simulink model "Vehicle_Control_CodeGen"  (R2024a)
settings: Solver=FixedStepAuto  StartTime=0.0  StopTime=10  RelTol=1e-3  EnableMultiTasking=on
undefined symbols (not defined in the file or in its folder): CAN, DiscIntNeverNeededParam, FD, Ion, Lithium
libraries: stmutilitieslib x28, simulink x21, stm32blockslib x10, canfdmsglib x6, dspstat3 x6, slpidlib x3, spsBatteryLib x2, spsControlledCurrentSourceLib x2, spsVoltageMeasurementLib x2, spspowerguiLib x2, stm32h7xxblockslib x2
(part 3 of 3)

== system Vehicle_Control_CodeGen/Variant Subsystem/CAN Forwarding ==
  In1 : Inport
  Out1 : Outport
  wires:
  In1/1 -> Out1/1

== system Vehicle_Control_CodeGen/Variant Subsystem/Simulation of Throttle Pedal ==
  note: Set sim time to 2154
  note: Throttle Input
  Constant1 : Constant  Value=50
  Constant25 : Constant  Value=100
  From File : FromFile  FileName=endurancedata.mat  SampleTime=0.1
  Manual Switch2 : ManualSwitch  CurrentSetting=0
  Product8 : Product
  Scope12 : Scope
  Out1 : Outport
  wires:
  From File/1 -> Product8/1  "Throttle"
  Constant1/1 -> Manual Switch2/1  "Throttle Percentage"
  Product8/1 -> Scope12/1, Manual Switch2/2  "Throttle"
  Constant25/1 -> Product8/2
  Manual Switch2/1 -> Out1/1

== system Vehicle_Control_CodeGen/Variant Subsystem1/Battery Model1 ==
  note: Delay increased to 3 x 0.01 second to test robustness. This is to simulate the delay of having voltage measurments sent to the VCU
  note: Battery Model is from SIM SCAPE Tool box. Uses a constant current drive to take the current request from controller and apply load to the battery
  Requested Current : Inport
  Battery1 : spsBatteryLib/Battery  BatType=Lithium-Ion  ShowTempParam=off  ThermalPreset=no  ShowAgeParam=off  NomV=532.8  NomQ=1152  SOC=85  Batt_Tr=5  PresetModel=on  MaxQ=1152  MinV=399.6  FullV=620.1723  Dis_rate=500.8696  R=0.004625  Normal_OP=1041.8087  expZone="[575.6296      56.59826]"  current=[6.5 13 32.5]  Units=Time  Tci=20  NomT=20  T2=-30  MaxQ2=4.8  FullV2=7.1  Normal_OP2=5.655  expZone2="[6.58           1]"  Rca=0.6  ti=2000  Dp=0  Neq0=0  Tsim=1e6  Ta1=25  Qeol=5.4*0.9  Reol=0.013333*1.2  Char_age=[2.3478, 3]  Dis_age=[2.3478, 10]  N1=1500  N2=10500  N3=1000  N4=1400  Ta2=45  N5=950
  Controlled Current Source1 : spsControlledCurrentSourceLib/Controlled Current Source  Initialize=on  Source_Type=AC  Amplitude=0  Phase=0  Frequency=0  Measurements=None
  Delay2 : Delay  DelayLength=5  InitialCondition=580
  Scope5 : Scope
  Voltage Measurement1 : spsVoltageMeasurementLib/Voltage Measurement  PhasorSimulation=off  OutputType=Complex  PSBequivalent=0
  powergui1 : spspowerguiLib/powergui  Priority=1  SimulationMode=Discrete  SampleTime=0.001  frequency=60  Iterations=50  frequencyindice=0  Pbase=100e6  ErrMax=1e-4  UnitsV=kV  UnitsW=MW  buscounter=0  FunctionMessages=off  echomessages=off  EnableUseOfTLC=off  CurrentSourceSwitches=off  DisableSnubberDevices=off  DisableRonSwitches=off  DisableVfSwitches=off  DisplayEquations=off  AutomaticDiscreteSolvers=off  SolverType=Tustin/Backward Euler (TBE)  Interpol=off  ExternalGateDelay=off  methode=off  Ts=100  x0status=blocks  SPID=on  SwTol=0  HookPort=off  NonlinearTolerance=1e-4  nMaxIteration=100  ContinueOnMaxIteration=off  RestoreLinks=warning  ResistiveCurrentMeasurement=off  Frange=[0:2:500]  Ylog=off  Xlog=on  ShowGrid=off  save=off  variable=ZData  structure=0  ZoomFFT=off  StartTime=0.0  cycles=1  DisplayStyle=1  fundamental=60  FreqAxis=off  MaxFrequency=1000  frequencyindicesteady=1  RmsSteady=1  display=off
  Scope : Outport
  Batt Out : Outport  Port=2
  wires:
  Voltage Measurement1/1 -> Delay2/1, Scope/1, Scope5/1  "BUS Voltage"
  Requested Current/1 -> Controlled Current Source1/1
  Delay2/1 -> Batt Out/1  "Batter Voltage"
  Battery1/1 -> ?
  connections:
  Voltage Measurement1/LConn1 -- Controlled Current Source1/RConn1 -- Battery1/LConn1
  Battery1/LConn2 -- Voltage Measurement1/LConn2 -- Controlled Current Source1/LConn1

== system Vehicle_Control_CodeGen/Variant Subsystem1/CAN Forwarding ==
  Can Sig : Inport
  Batt Out : Outport
  Scope : Outport  Port=2
  wires:
  Can Sig/1 -> Scope/1, Batt Out/1

== system Vehicle_Control_CodeGen/Power Forcasting/Variant Subsystem/CAN Forwarding ==
  CAN SOC : Inport
  Out1 : Outport
  wires:
  CAN SOC/1 -> Out1/1

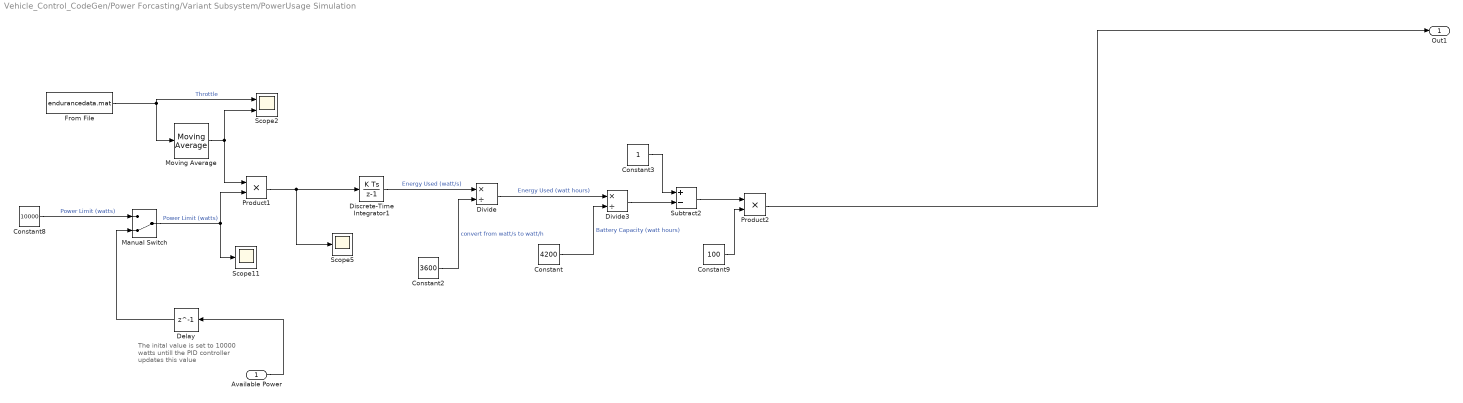
== system Vehicle_Control_CodeGen/Power Forcasting/Variant Subsystem/PowerUsage Simulation ==
  note: The inital value is set to 10000 watts untill the PID controller updates this value
  Available Power : Inport
  Constant : Constant  Value=4200
  Constant2 : Constant  Value=3600
  Constant3 : Constant
  Constant8 : Constant  Value=10000
  Constant9 : Constant  Value=100
  Delay : Delay  DelayLength=1  InitialCondition=10000
  Discrete-Time Integrator1 : DiscreteIntegrator  SampleTime=-1  ICPrevOutput=DiscIntNeverNeededParam  ICPrevScaledInput=DiscIntNeverNeededParam
  Divide : Product  Inputs=*/
  Divide3 : Product  Inputs=*/
  From File : FromFile  FileName=endurancedata.mat
  Manual Switch : ManualSwitch  CurrentSetting=0
  Moving Average : dspstat3/Moving Average  Method=Sliding window  ForgettingFactorPort=off  SpecifyWindowLength=on  WindowLength=1000  OverlapLength=999  AllowArbitraryInputLength=off  ForgettingFactor=0.9  SimulateUsing=Interpreted execution
  Product1 : Product
  Product2 : Product
  Scope11 : Scope
  Scope2 : Scope  NumInputPorts=2
  Scope5 : Scope
  Subtract2 : Sum  Inputs=+-
  Out1 : Outport
  wires:
  Moving Average/1 -> Scope2/2, Product1/1
  Constant8/1 -> Manual Switch/1  "Power Limit (watts)"
  Divide/1 -> Divide3/1  "Energy Used (watt hours)"
  Product1/1 -> Scope5/1, Discrete-Time Integrator1/1
  Divide3/1 -> Subtract2/2
  Delay/1 -> Manual Switch/2
  Subtract2/1 -> Product2/1
  Manual Switch/1 -> Scope11/1, Product1/2  "Power Limit (watts)"
  Constant9/1 -> Product2/2
  From File/1 -> Scope2/1, Moving Average/1  "Throttle"
  Discrete-Time Integrator1/1 -> Divide/1  "Energy Used (watt/s)"
  Constant3/1 -> Subtract2/1
  Constant2/1 -> Divide/2  "convert from watt/s to watt/h"
  Constant/1 -> Divide3/2  "Battery Capacity (watt hours)"
  Product2/1 -> Out1/1
  Available Power/1 -> Delay/1

== system Vehicle_Control_CodeGen/Power Forcasting/Variant Subsystem1/Code Gen, Wheel speed averaging and integration ==
  note: Filtering input to try and stop large changes in rate of change of distance traveled
  In2 : Inport
  In1 : Inport  Port=2
  Add2 : Sum
  Constant2 : Constant  Value=2
  Discrete-Time Integrator2 : DiscreteIntegrator  SampleTime=-1  ICPrevOutput=DiscIntNeverNeededParam  ICPrevScaledInput=DiscIntNeverNeededParam
  Divide : Product  Inputs=*/
  Moving Average1 : dspstat3/Moving Average  Method=Sliding window  ForgettingFactorPort=off  SpecifyWindowLength=on  WindowLength=1000  OverlapLength=999  AllowArbitraryInputLength=off  ForgettingFactor=0.9  SimulateUsing=Interpreted execution
  Scope : Scope
  Scope1 : Scope
  1 : Outport
  wires:
  Constant2/1 -> Divide/2
  Add2/1 -> Divide/1
  Divide/1 -> Discrete-Time Integrator2/1  "Average Speed"
  In2/1 -> Add2/1  "Right Wheel Speed"
  In1/1 -> Scope/1, Add2/2  "Left Wheel Speed"
  Discrete-Time Integrator2/1 -> Moving Average1/1  "Distance Traveled"
  Moving Average1/1 -> Scope1/1, 1/1

== system Vehicle_Control_CodeGen/Power Forcasting/Variant Subsystem1/Fake wheel speed from simulation ==
  note: Filtering input to try and stop large changes in rate of change of distance traveled
  Add2 : Sum
  Constant1 : Constant  Value=2
  Discrete-Time Integrator2 : DiscreteIntegrator  SampleTime=-1  ICPrevOutput=DiscIntNeverNeededParam  ICPrevScaledInput=DiscIntNeverNeededParam
  Discrete-Time Integrator3 : DiscreteIntegrator  SampleTime=-1  ICPrevOutput=DiscIntNeverNeededParam  ICPrevScaledInput=DiscIntNeverNeededParam
  Divide2 : Product  Inputs=*/
  From File1 : FromFile  FileName=simspeed.mat
  From File2 : FromFile  FileName=simspeed.mat
  From File3 : FromFile  FileName=simspeed.mat
  Manual Switch2 : ManualSwitch  CurrentSetting=0
  Moving Average1 : dspstat3/Moving Average  Method=Sliding window  ForgettingFactorPort=off  SpecifyWindowLength=on  WindowLength=1000  OverlapLength=999  AllowArbitraryInputLength=off  ForgettingFactor=0.9  SimulateUsing=Interpreted execution
  Moving Average2 : dspstat3/Moving Average  Method=Sliding window  ForgettingFactorPort=off  SpecifyWindowLength=on  WindowLength=1000  OverlapLength=999  AllowArbitraryInputLength=off  ForgettingFactor=0.9  SimulateUsing=Interpreted execution
  Scope : Scope
  Scope7 : Scope
  Scope8 : Scope  NumInputPorts=2
  Scope9 : Scope
  1 : Outport
  wires:
  Constant1/1 -> Divide2/2
  From File3/1 -> Add2/1  "Right Wheel Speed"
  Add2/1 -> Divide2/1
  Discrete-Time Integrator3/1 -> Moving Average2/1  "Distance Traveled"
  From File1/1 -> Scope7/1, Discrete-Time Integrator2/1  "vehicle Speed"
  Divide2/1 -> Discrete-Time Integrator3/1  "Average Speed"
  Discrete-Time Integrator2/1 -> Scope8/2, Moving Average1/1  "Distance Traveled"
  Moving Average2/1 -> Manual Switch2/1, Scope9/1  "Distance Traveled"
  Moving Average1/1 -> Scope8/1, Manual Switch2/2
  From File2/1 -> Scope/1, Add2/2  "Left Wheel Speed"
  Manual Switch2/1 -> 1/1

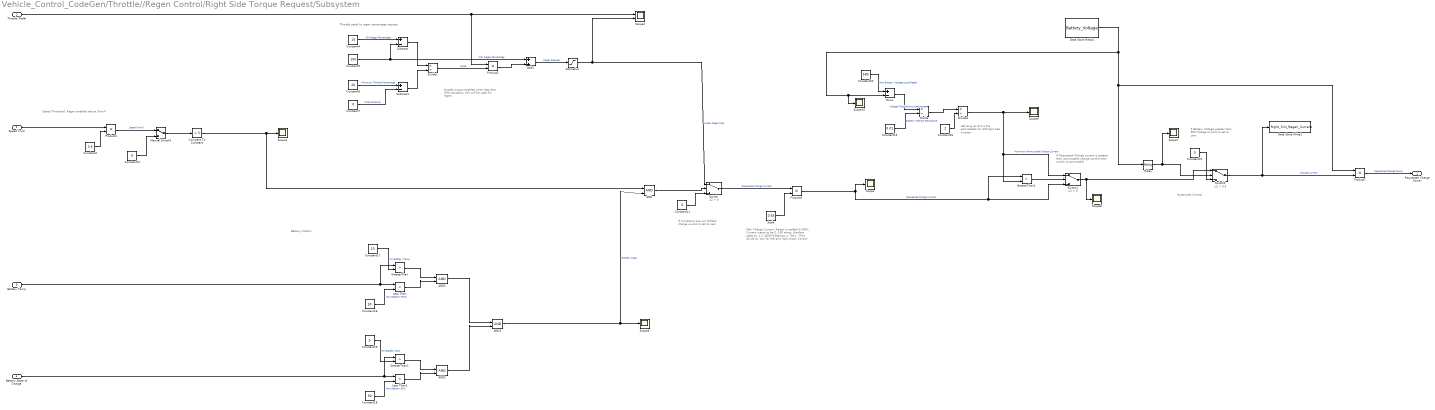
== system Vehicle_Control_CodeGen/Throttle//Regen Control/Right Side Torque Request/Subsystem ==
  note: Halveing as this is the permissable for left/right side inverter
  note: If Conditions are not fulfilled charge current is set to zero
  note: Throttle pedal to regen percentage request
  note: throttle output enabled when less then 20% actuation, this will be used for regen
  note: If Battery Voltage greater then 590 Charge Current is set to zero
  note: Speed Threshold, Regen enabled above 5km/h
  note: Max Charge Current, Regen is scalled 0-100%. Current wants to be 0 -130 amps, therfore scale by 1.3. 600V*130amps = 70kw, Then divide by two for left and right motor Control
  note: Hysterisies Control
  note: Battery Checks
  note: If Requested Charge current is greater then permissable charge current then switch to permisable
  Throttle Pedal : Inport
  Speed (m/s) : Inport  Port=2
  Battery Temp : Inport  Port=3
  Battery State of Charge : Inport  Port=4
  AND{,1..3} (4 alike) : Logic  IconShape=distinctive  AllPortsSameDT=off  OutDataTypeStr=boolean
  Add3 : Sum
  Compare To Constant : simulink/Logic and Bit Operations/Compare To Constant  relop=>  const=5  OutDataTypeStr=boolean
  Constant11 : Constant  Value=0
  Constant12 : Constant  Value=6
  Constant15 : Constant  Value=0.01
  Constant16 : Constant  Value=50
  Constant17 : Constant  Value=10
  Constant18 : Constant  Value=90
  Constant19 : Constant  Value=5
  Constant2 : Constant  Value=3.6
  Constant20 : Constant  Value=580
  Constant21 : Constant  Value=0
  Constant26 : Constant  Value=2
  Constant4 : Constant  Value=10
  Constant5 : Constant  Value=100
  Constant6 : Constant  Value=20
  Constant7 : Constant  Value=0
  Data Store Read1 : DataStoreRead  DataStoreName=Battery_Voltage  IndexOptions=Index vector (dialog)  Indices=1  OutputSizes=1
  Data Store Write1 : DataStoreWrite  DataStoreName=Right_Sim_Regen_Current  IndexOptions=Index vector (dialog)  Indices=1  OutputSizes=1
  Divide : Product  Inputs=*/
  Divide1 : Product  Inputs=*/
  Divide4 : Product  Inputs=*/
  GreaterThan : RelationalOperator  Operator=>  OutDataTypeStr=boolean  RndMeth=Simplest  InputSameDT=off
  GreaterThan1 : RelationalOperator  Operator=>  OutDataTypeStr=boolean  RndMeth=Simplest  InputSameDT=off
  GreaterThan2 : RelationalOperator  Operator=>  OutDataTypeStr=boolean  RndMeth=Simplest  InputSameDT=off
  Less Than : RelationalOperator  Operator=<  OutDataTypeStr=boolean  RndMeth=Simplest  InputSameDT=off
  Less Than1 : RelationalOperator  Operator=<  OutDataTypeStr=boolean  RndMeth=Simplest  InputSameDT=off
  Manual Switch1 : ManualSwitch
  Minus : Sum  Inputs=+-
  Product{1..2,4,7} (4 alike) : Product
  Relay : Relay  OnSwitchValue=590  OffSwitchValue=585  OnOutputValue=0  OffOutputValue=1
  Saturation : Saturate  UpperLimit=100  LowerLimit=0
  Scale : Constant  Value=0.65
  Scope{,1,3,7..9,15} (7 alike) : Scope
  Scope2 : Scope  NumInputPorts=2
  Subtract : Sum  Inputs=+-
  Subtract1 : Sum  Inputs=+-
  Switch : Switch  Criteria=u2 > Threshold  SaturateOnIntegerOverflow=off  InputSameDT=off
  Switch1 : Switch  Criteria=u2 > Threshold  SaturateOnIntegerOverflow=off  InputSameDT=off
  Switch2 : Switch  Criteria=u2 > Threshold  Threshold=0.5  SaturateOnIntegerOverflow=off  InputSameDT=off
  Requested Charge Power : Outport
  wires:
  AND3/1 -> Scope3/1, AND/2  "Battery Logic"
  Constant21/1 -> Switch2/3
  Constant5/1 -> Subtract/2, Add3/1  "Max Regen Percentage"
  Relay/1 -> Switch2/2, Scope7/1
  Manual Switch1/1 -> Compare To Constant/1
  Constant2/1 -> Product1/2
  Constant18/1 -> Less Than1/2  "Max Battery SOC"
  Constant20/1 -> Minus/1  "Max Battery Voltage using Regen"
  Compare To Constant/1 -> AND/1, Scope1/1
  Subtract1/1 -> Divide1/2
  Divide1/1 -> Product2/2  "Slope"
  Constant12/1 -> Manual Switch1/2
  Scale/1 -> Product4/2
  Constant17/1 -> GreaterThan/2  "Min Battery Temp"
  Constant16/1 -> Less Than/2  "Max Battery temp"
  Throttle Pedal/1 -> Product2/1, Scope2/1
  AND2/1 -> AND3/2
  Battery Temp/1 -> GreaterThan/1, Less Than/1
  Minus/1 -> Divide/1  "Voltage Threshold to overcharge"
  Less Than1/1 -> AND2/2
  Product2/1 -> Add3/2
  Switch1/1 -> Switch2/1, Scope8/1
  GreaterThan/1 -> AND1/1
  Product4/1 -> Scope/1, Switch1/3, GreaterThan2/1  "Requested Charge Current"
  Battery State of Charge/1 -> GreaterThan1/1, Less Than1/1
  AND/1 -> Switch/2
  Divide/1 -> Divide4/1
  Switch2/1 -> Data Store Write1/1, Product7/2  "Charge Current"
  Constant15/1 -> Divide/2  "Battery Internal Resistance"
  Constant19/1 -> GreaterThan1/2  "Min Battery SOC"
  AND1/1 -> AND3/1
  Constant7/1 -> Subtract1/2  "Intial distance"
  Subtract/1 -> Divide1/1
  GreaterThan2/1 -> Switch1/2
  Divide4/1 -> GreaterThan2/2, Switch1/1, Scope9/1  "Maximum Permissable Charge Current"
  Less Than/1 -> AND1/2
  Switch/1 -> Product4/1  "Requested Charge Current"
  Product1/1 -> Manual Switch1/1  "Speed (km/h)"
  Add3/1 -> Saturation/1  "Regen Request"
  Constant11/1 -> Switch/3
  GreaterThan1/1 -> AND2/1
  Data Store Read1/1 -> Scope15/1, Minus/2, Product7/1, Relay/1
  Constant26/1 -> Divide4/2
  Saturation/1 -> Switch/1, Scope2/2  "Linear Regen Map"
  Constant6/1 -> Subtract1/1  "Minimum Throttle Percentage"
  Constant4/1 -> Subtract/1  "Min Regen Percentage"
  Product7/1 -> Requested Charge Power/1  "Requested Charge Power"
  Speed (m/s)/1 -> Product1/1

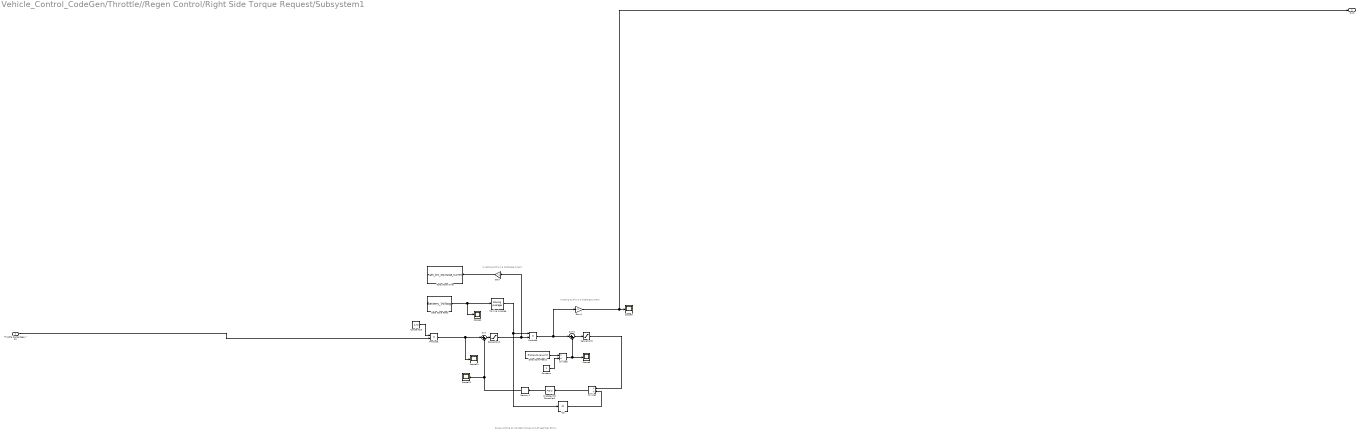
== system Vehicle_Control_CodeGen/Throttle//Regen Control/Right Side Torque Request/Subsystem1 ==
  note: Power Limiting to maintatin Power Limit of Less then 80 Kw
  note: Inverting as this is a discharge current
  note: Inverting as this is a discharge current
  Throttle Percentage > 20 : Inport
  Constant : Constant  Value=2
  Constant23 : Constant  Value=0.75
  Data Store Read : DataStoreRead  DataStoreName=Battery_Voltage  IndexOptions=Index vector (dialog)  Indices=1  OutputSizes=1
  Data Store Read2 : DataStoreRead  DataStoreName=Global_Power_Limit  IndexOptions=Index vector (dialog)  Indices=1  OutputSizes=1
  Data Store Write : DataStoreWrite  DataStoreName=Right_Sim_Discharge_Current  IndexOptions=Index vector (dialog)  Indices=1  OutputSizes=1
  Discrete PID Controller1 : slpidlib/PID Controller  Controller=PID  Form=Parallel  TimeDomain=Discrete-time  UseExternalTs=off  SampleTime=-1  IntegratorMethod=Forward Euler  FilterMethod=Forward Euler  ControllerParametersSource=internal  P=0.000544217300579932  I=0.544217300579932  UseKiTs=on  D=0  UseExternalDerivativeSource=off  N=100  UseFilter=on  TunerSelectOption=Transfer Function Based (PID Tuner App)  InitialConditionSource=internal  InitialConditionForIntegrator=10  InitialConditionForFilter=0  DifferentiatorICPrevScaledInput=0  ExternalReset=none  TrackingMode=off  Kt=1  LimitOutput=off  SatLimitsSource=internal  UpperSaturationLimit=inf  LowerSaturationLimit=-inf  LinearizeAsGain=off  AntiWindupMode=none  Kb=1  LimitIntegrator=off  UpperIntegratorSaturationLimit=inf  LowerIntegratorSaturationLimit=-inf  POutMin=[]  POutMax=[]  IOutMin=[]  IOutMax=[]  DOutMin=[]  DOutMax=[]  NOutMin=[]  NOutMax=[]  SumOutMin=[]  SumOutMax=[]  SaturationOutMin=[]  SaturationOutMax=[]  PParamMin=[]  PParamMax=[]  IParamMin=[]  IParamMax=[]  DParamMin=[]  DParamMax=[]  NParamMin=[]  NParamMax=[]  KbParamMin=[]  KbParamMax=[]  KtParamMin=[]  KtParamMax=[]  KbOutMin=[]  KbOutMax=[]  KtOutMin=[]  KtOutMax=[]  IntegratorOutMin=[]  IntegratorOutMax=[]  FilterOutMin=[]  FilterOutMax=[]  SumI1OutMin=[]  SumI1OutMax=[]  SumI2OutMin=[]  SumI2OutMax=[]  SumI3OutMin=[]  SumI3OutMax=[]  SumI4OutMin=[]  SumI4OutMax=[]  SumDOutMin=[]  SumDOutMax=[]  DifferentiatorOutMin=[]  DifferentiatorOutMax=[]  FilterDiffOutCoefMin=[]  FilterDiffOutCoefMax=[]  ReciprocalOutMin=[]  ReciprocalOutMax=[]  SumDenOutMin=[]  SumDenOutMax=[]  SumNumOutMin=[]  SumNumOutMax=[]  DivideOutMin=[]  DivideOutMax=[]  UdiffTsProdOutMin=[]  UdiffTsProdOutMax=[]  NTsProdOutMin=[]  NTsProdOutMax=[]  UintegralTsProdOutMin=[]  UintegralTsProdOutMax=[]  UngainTsProdOutMin=[]  UngainTsProdOutMax=[]  ClampingZeroOutDataTypeStr=Inherit: Inherit via back propagation  ClampingZeroOutMin=[]  ClampingZeroOutMax=[]  FilterDenConstantOutDataTypeStr=Inherit: Inherit via back propagation  FilterDenConstantOutMin=[]  FilterDenConstantOutMax=[]  PCopyOutDataTypeStr=Inherit: Inherit via back propagation  PCopyOutMin=[]  PCopyOutMax=[]  NCopyOutDataTypeStr=Inherit: Inherit via back propagation  NCopyOutMin=[]  NCopyOutMax=[]  IntegratorContinuousStateAttributes=''  IntegratorStateMustResolveToSignalObject=off  IntegratorRTWStateStorageClass=Auto  FilterContinuousStateAttributes=''  FilterStateMustResolveToSignalObject=off  FilterRTWStateStorageClass=Auto  ParallelPVariant=InternalParameters  IdealPVariant=Disabled  IVariant=InternalParameters  DVariant=InternalParameters  IntegratorVariant=Discrete  SatVariant=Disabled  AWVariant=Passthrough  PCopyVariant=Disabled  TRVariant=Disabled  FdbkBlocksVariant=Forward  IdealPFdbkVariant=Disabled  SatFdbkVariant=Disabled  DerivativeFilterVariant=ForwardEulerFilter  NVariant=InternalParameters  NCopyVariant=Disabled  FilterICVariant=InternalICsFilter  IntegratorICVariant=InternalICs  ExternalResetVariant=Disabled  TRSumVariant=Passthrough  SumFdbkVariant=Disabled  SumVariant=Sum_PID  TsampFilterVariant=InternalTs  TsampNgainVariant=Passthrough  TsampIntegralVariant=Disabled_SignalSpec  ExternalSaturationOutDataTypeStr=Inherit: Same as second input  DerivativeSourceVariant=ErrorSignal
      settings: LibrarySourceBlock=simulink/Discrete/Discrete PID Controller
  Divide2 : Product  Inputs=*/
  Divide3 : Product  Inputs=*/
  Gain : Gain  Gain=-1
  Gain1 : Gain  Gain=-1
  IC2 : InitialCondition  Value=600
  Memory1 : Memory  InitialCondition=14  InheritSampleTime=on
  Moving Average : dspstat3/Moving Average  Method=Sliding window  ForgettingFactorPort=off  SpecifyWindowLength=on  WindowLength=10  OverlapLength=9  AllowArbitraryInputLength=off  ForgettingFactor=0.9  SimulateUsing=Interpreted execution
  Product5 : Product
  Product6 : Product
  Saturation3 : Saturate  UpperLimit=inf  LowerLimit=0
  Saturation5 : Saturate  UpperLimit=inf  LowerLimit=0
  Scope{4..6,10,12} (5 alike) : Scope
  Sum : Sum  Inputs=|+-
  Sum1 : Sum  Inputs=|+-
  Out1 : Outport
  wires:
  Data Store Read/1 -> Scope4/1, Moving Average/1
  Memory1/1 -> Sum/2, Scope12/1
  Gain/1 -> Data Store Write/1
  Product5/1 -> Sum1/1, Gain1/1  "Requested Discharge Power"
  Sum/1 -> Saturation5/1
  IC2/1 -> Divide2/2
  Sum1/1 -> Saturation3/1
  Gain1/1 -> Out1/1, Scope5/1
  Divide3/1 -> Scope6/1, Sum1/2
  Product6/1 -> Sum/1, Scope10/1  "Current Request (0-75amps)"
  Saturation5/1 -> Gain/1, Product5/2
  Divide2/1 -> Discrete PID Controller1/1  "Current Error"
  Discrete PID Controller1/1 -> Memory1/1
  Throttle Percentage > 20/1 -> Product6/2
  Constant/1 -> Divide3/2
  Data Store Read2/1 -> Divide3/1
  Constant23/1 -> Product6/1
  Moving Average/1 -> IC2/1, Product5/1
  Saturation3/1 -> Divide2/1  "Power Error"
